simulink model "LSTMTestEnviroment"  (R2024a)
settings: Solver=VariableStepAuto  StartTime=0.0  StopTime=86400  RelTol=1e-3
undefined symbols (not defined in the file or in its folder): muX, sigmaX
libraries: deeplib x1
settings Model: Creator=Connor du Toit  LastModifiedBy=Connor du Toit

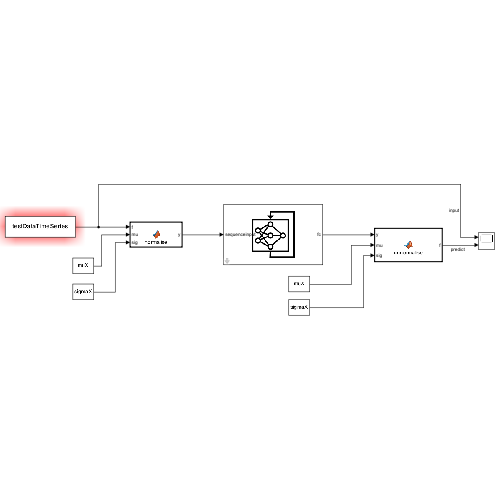
[thumbnail: Simulink's stored preview of the top-level diagram]
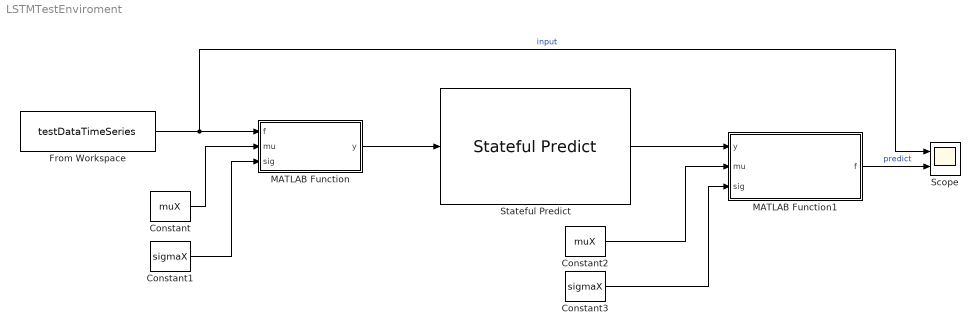
== system LSTMTestEnviroment ==
  Constant : Constant  Value=muX
  Constant1 : Constant  Value=sigmaX
  Constant2 : Constant  Value=muX
  Constant3 : Constant  Value=sigmaX
  From Workspace : FromWorkspace  VariableName=testDataTimeSeries  SampleTime=1
  MATLAB Function : MATLAB Function  TreatAsAtomicUnit=on
  MATLAB Function1 : MATLAB Function  TreatAsAtomicUnit=on
  Scope : Scope  NumInputPorts=2
  Stateful Predict : deeplib/Stateful Predict  Network=Network from MAT-file  NetworkFunction=untitled  NetworkFilePath=C:\Users\Connor du Toit\Documents\Research Project\LSTM Training\NET_LSTM_2023_irradiance.mat  InputDataFormats={ 'sequenceinput', 'TCB' }  SampleTime=1  ForceInterpretedSim=off  EnableDLNetwork=on  LastKnownNetworkFilePath='C:\Users\Connor du Toit\Documents\Research Project\LSTM Training\NET_LSTM_2023_irradiance.mat'  LastKnownNetworkTimeStamp=739538.401504629640839993953704833984375
  wires:
  MATLAB Function/1(y) -> Stateful Predict/1
  From Workspace/1 -> Scope/1, MATLAB Function/1(f)  "input"
  Stateful Predict/1 -> MATLAB Function1/1(y)
  Constant/1 -> MATLAB Function/2(mu)
  Constant1/1 -> MATLAB Function/3(sig)
  Constant2/1 -> MATLAB Function1/2(mu)
  Constant3/1 -> MATLAB Function1/3(sig)
  MATLAB Function1/1(f) -> Scope/2  "predict"

== matlab function LSTMTestEnviroment/MATLAB Function1 ==
  data: y input; f output; mu input; sig input
function f = unnormalise(y, mu, sig)

f = (y*sig) + mu;

== matlab function LSTMTestEnviroment/MATLAB Function ==
  data: f input; y output; mu input; sig input
function y = normalise(f, mu, sig)

y = (f - mu)/sig;
